simulink model "TestStabilityController"  (R2022b)
settings: Solver=FixedStepAuto  StartTime=0.0  StopTime=50.0  FixedStep=simulator.TimeStep  RelTol=1e-3
undefined symbols (not defined in the file): simulator
settings Model: Creator=At  LastModifiedBy=ateay
settings SolverCC: ConcurrentTasks=on  AlgebraicLoopSolver=TrustRegion  InsertRTBMode=Never (minimum delay)
settings DataIOCC: ReturnWorkspaceOutputs=off
settings DebuggingCC: UnconnectedInputMsg=warning  UnconnectedOutputMsg=warning  UnconnectedLineMsg=warning  SFMachineParentedDataDiag=warning  ArithmeticOperatorsInVariantConditions=warning
settings ModelReferenceCC: EnableRefExpFcnMdlSchedulingChecks=on
settings SFSimCC: SimUseLocalCustomCode=off  CustomCodeUndefinedFunction=UseInterfaceOnly
settings RTWCC: RTWUseLocalCustomCode=off
settings CodeAppCC: StateflowObjectComments=on

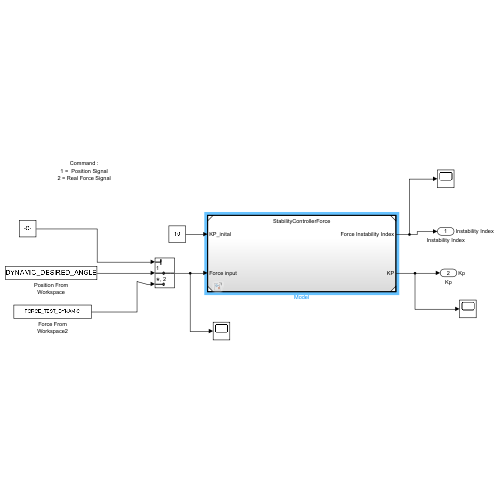
[thumbnail: Simulink's stored preview of the top-level diagram]
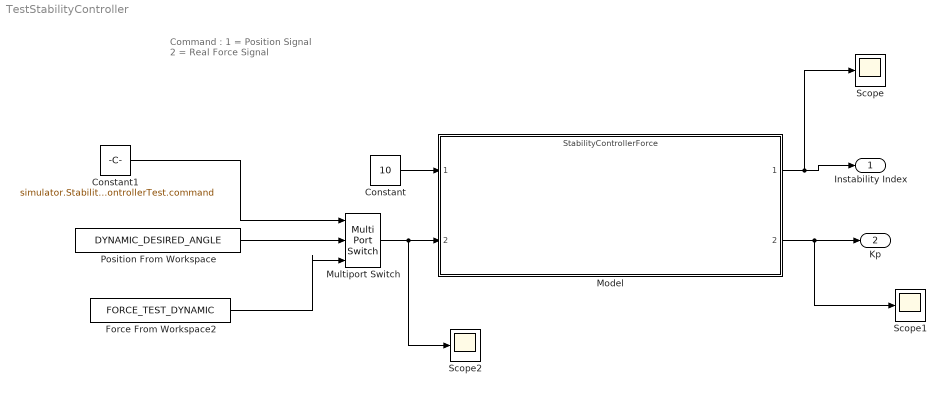
== system TestStabilityController ==
  note: Command :
      | 1 =  Position Signal
      | 2 = Real Force Signal
  Constant : Constant  Value=10
  Constant1 : Constant  Value=simulator.StabilityControllerTest.command
  Force From Workspace2 : FromWorkspace  VariableName=FORCE_TEST_DYNAMIC
  Model : ModelReference  ModelNameDialog=StabilityControllerForce.slx  SimulationMode=Normal  ModelReferenceVersion=13.0
  Multiport Switch : MultiPortSwitch  Inputs=2  SaturateOnIntegerOverflow=off  InputSameDT=off
  Position From Workspace : FromWorkspace  VariableName=DYNAMIC_DESIRED_ANGLE
  Scope : Scope
  Scope1 : Scope
  Scope2 : Scope
  Instability Index : Outport  SignalName=Instability Index
  Kp : Outport  Port=2  SignalName=Kp
  wires:
  Constant/1 -> Model/1
  Model/2 -> Scope1/1, Kp/1
  Model/1 -> Scope/1, Instability Index/1
  Constant1/1 -> Multiport Switch/1
  Position From Workspace/1 -> Multiport Switch/2
  Force From Workspace2/1 -> Multiport Switch/3
  Multiport Switch/1 -> Scope2/1, Model/2
